simulink model "ProductMultiple"  (R2017b)
settings: Solver=ode3  StartTime=0.0  StopTime=10.0  FixedStep=0.200000  RelTol=1e-3
settings Model: Creator=hbourbou  LastModifiedBy=hbourbou
settings OptimizationCC: LifeSpan=inf
settings DebuggingCC: SFExecutionAtInitializationDiag=none
settings HardwareCC: ProdBitPerSizeT=32  ProdBitPerPtrDiffT=32  ProdWordSize=32  ProdHWDeviceType=Specified
settings CodeAppCC: StateflowObjectComments=on

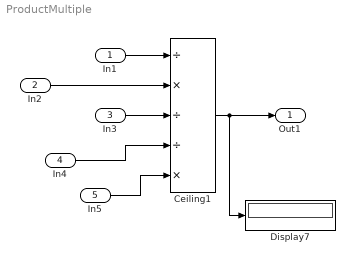
== system ProductMultiple ==
  In1 : Inport
  In2 : Inport  Port=2
  In3 : Inport  Port=3
  In4 : Inport  Port=4
  In5 : Inport  Port=5
  Ceiling1 : Product  Inputs=/*//*  RndMeth=Ceiling
  Display7 : Display
  Out1 : Outport
  wires:
  In1/1 -> Ceiling1/1
  In2/1 -> Ceiling1/2
  In3/1 -> Ceiling1/3
  In4/1 -> Ceiling1/4
  In5/1 -> Ceiling1/5
  Ceiling1/1 -> Out1/1, Display7/1
